simulink model "rlwatertankReward"  (R2022b)
settings: Solver=FixedStepAuto  StartTime=0.0  StopTime=10  FixedStep=0.01  RelTol=1e-3  EnableMultiTasking=on
undefined symbols (not defined in the file or in its folder): DiscIntNeverNeededParam
settings Model: DataDictionary=BusSystem.sldd  Creator=The MathWorks, Inc.  LastModifiedBy=robert
settings SolverCC: AlgebraicLoopSolver=TrustRegion
settings DataIOCC: LimitDataPoints=on  SaveOutput=off  ReturnWorkspaceOutputs=off  SignalLoggingName=logsOut
settings OptimizationCC: ExpressionDepthLimit=2147483647  InitFltsAndDblsToZero=on  LifeSpan=inf
settings DebuggingCC: SaveWithParameterizedLinksMsg=none  UnderspecifiedInitializationDetection=Classic  MergeDetectMultiDrivingBlocksExec=none  SignalResolutionControl=TryResolveAllWithWarning  MultiTaskDSMMsg=warning  FcnCallInpInsideContextMsg=warning  UnconnectedInputMsg=warning  UnconnectedOutputMsg=warning  UnconnectedLineMsg=warning  AllowSymbolicDim=off  StateNameClashWarn=warning  SFUnexpectedBacktrackingDiag=warning  SFNoUnconditionalDefaultTransitionDiag=warning  SFExecutionAtInitializationDiag=none  SFMachineParentedDataDiag=warning  ArithmeticOperatorsInVariantConditions=warning
settings HardwareCC: ProdBitPerPointer=32  ProdBitPerSizeT=32  ProdBitPerPtrDiffT=32  ProdLargestAtomicFloat=None  ProdIntDivRoundTo=Undefined  ProdEndianess=Unspecified  ProdWordSize=32  ProdHWDeviceType=Specified
settings ModelReferenceCC: EnableRefExpFcnMdlSchedulingChecks=on  PropagateSignalLabelsOutOfModel=off
settings SFSimCC: SimUseLocalCustomCode=off  CustomCodeUndefinedFunction=UseInterfaceOnly
settings RTWCC: RTWUseLocalCustomCode=off  DLArmComputeVersion=19.05
settings CodeAppCC: StateflowObjectComments=on
settings GRTTargetCC: TargetFcnLib=ansi_tfl_tmw.mat  TargetLangStandard=C89/C90 (ANSI)  CombineOutputUpdateFcns=off  GRTInterface=on
settings ConfigComp: CovMetricSettings=dw  CovSaveCumulativeToWorkspaceVar=on  CovSaveSingleToWorkspaceVar=on  CovExternalEMLEnable=off

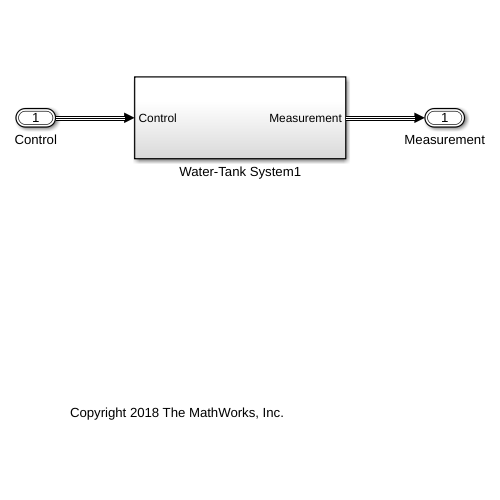
[thumbnail: Simulink's stored preview of the top-level diagram]
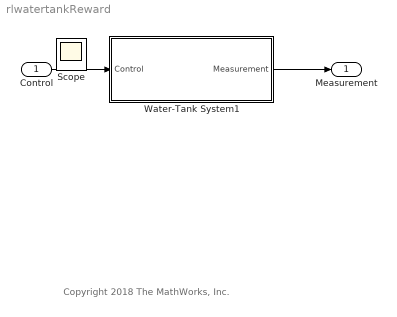
== system rlwatertankReward ==
  note: Copyright 2018 The MathWorks, Inc.
  Control : Inport  OutDataTypeStr=Bus: Control
  Water-Tank System1 : Subsystem
  Measurement : Outport  OutDataTypeStr=Bus: slBus3
  Scope : Scope
  wires:
  Control/1 -> Water-Tank System1/1(Control)
  Water-Tank System1/1(Measurement) -> Measurement/1

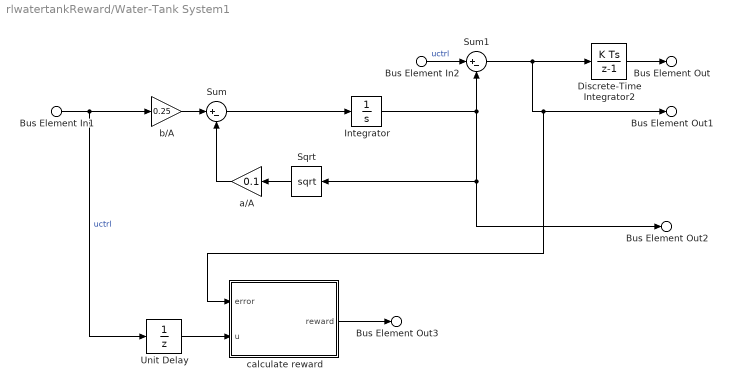
== system rlwatertankReward/Water-Tank System1 ==
  Bus Element In1 : Inport  PortName=Control  Element=uctrl
  Bus Element In2 : Inport  PortName=Control  Element=ref
  Discrete-Time Integrator2 : DiscreteIntegrator  SampleTime=-1  LowerSaturationLimit=0  ICPrevOutput=DiscIntNeverNeededParam  ICPrevScaledInput=DiscIntNeverNeededParam
  Integrator : Integrator  LimitOutput=on  LowerSaturationLimit=0
  Sqrt : Sqrt  OutputSignalType=real
  Sum : Sum  Inputs=|+-  SaturateOnIntegerOverflow=on
  Sum1 : Sum  Inputs=|+-
  Unit Delay : UnitDelay  SampleTime=-1  HasFrameUpgradeWarning=on
  a/A : Gain  Gain=0.1  SaturateOnIntegerOverflow=on  OutDataTypeStr=Inherit: Same as input  ParamDataTypeStr=Inherit: Same as input
  b/A : Gain  Gain=0.25  SaturateOnIntegerOverflow=on  OutDataTypeStr=Inherit: Same as input  ParamDataTypeStr=Inherit: Same as input
  calculate reward : Subsystem
  Bus Element Out3 : Outport  PortName=Measurement  Element=Reward
  Bus Element Out : Outport  PortName=Measurement  Element=errorIntegral
  Bus Element Out1 : Outport  PortName=Measurement  Element=error
  Bus Element Out2 : Outport  PortName=Measurement  Element=Height
  wires:
  a/A/1 -> Sum/2
  Sum/1 -> Integrator/1
  Sqrt/1 -> a/A/1
  Bus Element In1/1 -> Unit Delay/1, b/A/1  "uctrl"
  b/A/1 -> Sum/1
  Bus Element In2/1 -> Sum1/1  "uctrl"
  Sum1/1 -> calculate reward/1(error), Bus Element Out1/1, Discrete-Time Integrator2/1
  Discrete-Time Integrator2/1 -> Bus Element Out/1
  Integrator/1 -> Bus Element Out2/1, Sqrt/1, Sum1/2
  calculate reward/1(reward) -> Bus Element Out3/1
  Unit Delay/1 -> calculate reward/2(u)

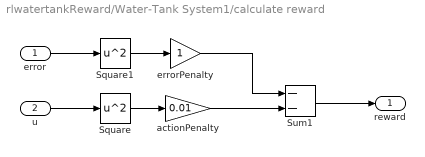
== system rlwatertankReward/Water-Tank System1/calculate reward ==
  error : Inport
  u : Inport  Port=2
  Square : Math  Operator=square
  Square1 : Math  Operator=square
  Sum1 : Sum  Inputs=--  OutDataTypeStr=double
  actionPenalty : Gain  Gain=0.01
  errorPenalty : Gain
  reward : Outport  VectorParamsAs1DForOutWhenUnconnected=off
  wires:
  Square1/1 -> errorPenalty/1
  errorPenalty/1 -> Sum1/1
  actionPenalty/1 -> Sum1/2
  Square/1 -> actionPenalty/1
  u/1 -> Square/1
  error/1 -> Square1/1
  Sum1/1 -> reward/1
